simulink model "FilterModel"  (R2020b)
settings: Solver=VariableStepAuto  StartTime=0.0  StopTime=10  RelTol=1e-3
settings Model: Creator=BIDITA PAUL  LastModifiedBy=BIDITA PAUL

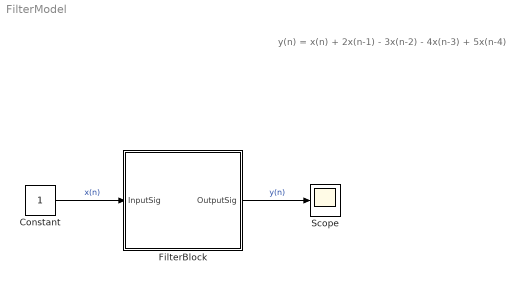
== system FilterModel ==
  note: y(n) = x(n) + 2x(n-1) - 3x(n-2) - 4x(n-3) + 5x(n-4)
  Constant : Constant
  FilterBlock : Subsystem  TreatAsAtomicUnit=on
  Scope : Scope
  wires:
  Constant/1 -> FilterBlock/1(InputSig)  "x(n)"
  FilterBlock/1(OutputSig) -> Scope/1  "y(n)"

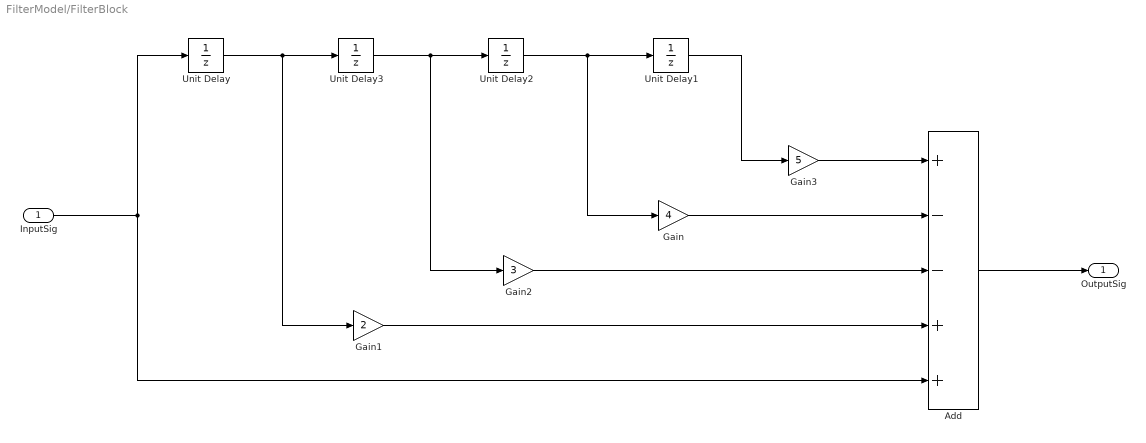
== system FilterModel/FilterBlock ==
  InputSig : Inport
  Add : Sum  Inputs=+--++
  Gain : Gain  Gain=4
  Gain1 : Gain  Gain=2
  Gain2 : Gain  Gain=3
  Gain3 : Gain  Gain=5
  Unit Delay{,1..3} (4 alike) : UnitDelay  SampleTime=-1  HasFrameUpgradeWarning=on
  OutputSig : Outport
  wires:
  Unit Delay/1 -> Gain1/1, Unit Delay3/1
  Gain2/1 -> Add/3
  Unit Delay1/1 -> Gain3/1
  Unit Delay2/1 -> Gain/1, Unit Delay1/1
  Gain/1 -> Add/2
  Unit Delay3/1 -> Gain2/1, Unit Delay2/1
  Gain3/1 -> Add/1
  Gain1/1 -> Add/4
  InputSig/1 -> Unit Delay/1, Add/5
  Add/1 -> OutputSig/1
